simulink model "Audio_BPSK"  (R2021b)
settings: Solver=VariableStepAuto  StartTime=0.0  StopTime=2  RelTol=1e-3
model workspace (MAT data in the model file):
  Fcarrier = 8000
  Fsampling = 48000
  Tsymbol = 0.0005
  beta = 0.5
  costas_alpha = 0.1
  costas_coeffs = [0.078989 0.085868 0.091518 0.095721 0.098311 0.099186 0.098311 0.095721 0.09151 0.085868 0.078989]
  filterSpan = 2
  gardner_Ki = -0.000314099
  gardner_Kp = -0.0282632
  int_presc = 0.6
  preamble = [1 1 1 -1 1]
  preambleLength = 5
  samplesPerSymbol = 24
  symbolsPerFrame = 8
undefined symbols (not defined in the file or in its folder): doppler, fdesignblkfcn, gcbh
libraries: commutil2 x3, commfilt2 x2, simulink x1, commsink2 x1, impairlib x1, commrandsrc3 x1, commchan3 x1
settings Model: SimulationMode=accelerator  PacingRate=0.071000  Creator=asiem  LastModifiedBy=asiem

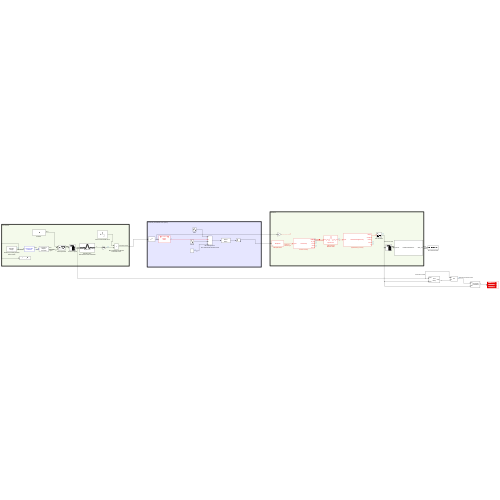
[thumbnail: Simulink's stored preview of the top-level diagram]
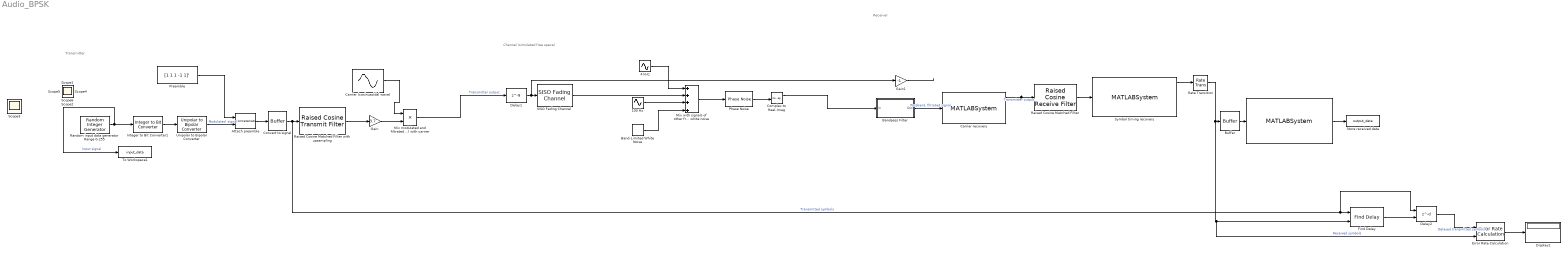
== system Audio_BPSK ==
  note: Receiver
  note: Channel (simulated free space)
  note: Transmitter
  " " : MATLABSystem  System=DataFramesDetector  buffer_length=512  preamble=[ 1, 1, 1, -1, 1 ]  data_frames_length=8  SimulateUsing=Interpreted execution
      mask Type: DataFramesDetector
      mask Display:
      | disp('DataFramesDetector');
      | port_label('input',1,'symbols');
      | port_label('output',1,'data_out');
  100 Hz : Sin  Amplitude=0.6  Bias=0.120  Frequency=100*2*pi  Phase=3*pi/4  SampleTime=1/48000
  "4 kHz " : Sin  Amplitude=0.3  Frequency=3000*2*pi  Phase=pi/3  SampleTime=1/48000
  Attach preamble : Concatenate  Mode=Multidimensional array
  Band-Limited White Noise : simulink/Sources/Band-Limited White Noise  Cov=[0.00000005]  Ts=1/Fsampling  seed=[23341]
  Bandpass Filter : Subsystem  DialogController=fdesignblkfcn  InitFcn=fdesignblkfcn(gcbh, {'InitFcn'});  mask(Bandpass Filter){}
      mask help: Design a bandpass filter
      settings: CopyFcn=fdesignblkfcn(gcbh, {'CopyFcn'});
      mask Help: helpview(mapfilelocation('dsp'), 'dspbandpassfilter');
      mask Display: disp('Bandpass');
  Buffer : Buffer  N=512  OutputFrames=off
  Carrier (cosinusoidal wave) : Sin  Frequency=Fcarrier*2*pi  Phase=pi/2 + pi/3  SampleTime=1/Fsampling
  Carrier recovery : MATLABSystem  System=CostasLoop  alpha=costas_alpha  beta=costas_alpha * costas_alpha / 4  lpf_coeffs=costas_coeffs  Fc=Fcarrier  Fs=Fsampling  REF_PERIOD=1e6 / Fcarrier  SAMPLE_PERIOD=1e6 / Fsampling  intgralf=int_presc * costas_alpha / (1e6 / Fcarrier)  SimulateUsing=Interpreted execution
      mask Type: CostasLoop
      mask Display:
      | disp('CostasLoop');
      | port_label('input',1,'input');
      | port_label('output',1,'S_I');
      | port_label('output',2,'S_Q');
      | port_label('output',3,'lock');
      | port_label('output',4,'ask');
      | port_label('output',5,'error');
  Complex to Real-Imag : ComplexToRealImag
  Convert to signal : Buffer  N=1  OutputFrames=off
  Delay1 : Delay  DelayLength=9  InputProcessing=Columns as channels (frame based)
  Delay2 : Delay  DelayLengthSource=Input port  DelayLength=3  InputProcessing=Columns as channels (frame based)
      settings: InputPortMap=u0,p1
  Display2 : Display
  Error Rate Calculation : commsink2/Error Rate Calculation  N=0  st_delay=0  cp_mode=Entire frame  subframe=[]  PMode=Port  WsName=ErrorVec  RsMode2=off  stop=off  numErr=100  maxBits=1e6
  Find Delay : commutil2/Find Delay  corrLength=20  chgSigOP=off  stopUpdate=off  numConstDelay=3
      settings: SourceProductBaseCode=CM
  Gain : Gain  Gain=3.7
  Gain1 : Gain  Gain=-1
  Integer to Bit Converter1 : commutil2/Integer to Bit Converter  nbits=symbolsPerFrame  signedInputValues=Unsigned  bitOrder=MSB first  outDtype=Inherit via internal rule
  Mix modulated and filtrated signal with carrier : Product
  Mix with signals of other frequencies and white noise : Sum  Inputs=++++
  Phase Noise : impairlib/Phase Noise  Level=-25  FrequencyOffset=3  SampleRate=Fsampling  RandomStream=mt19937ar with seed  Seed=32  SimulateUsing=Interpreted execution
      settings: SourceProductBaseCode=CM,AM,SX
  Preamble : Constant  Value=[1 1 1 -1 1]'  VectorParams1D=off
  "Raised Cosine Matched Filter " : commfilt2/Raised Cosine Receive Filter  filtType=Square root  R=beta  filtSpan=filterSpan  N=samplesPerSymbol  downFactor=1  downOffset=0  filterGain=1/2  InputProcessing=Columns as channels (frame based)  RateOptions=Allow multirate processing  framing=Mute  checkCoeff=on  variableName=rcRxFilt  currentFiltSpan=10  D=5  inputOffset=0  sampMode=Mute  saveAsFlag=0  rateMode=Downsampling  checkGain=Normalized  launchFVT=on  roundingMode=Floor  overflowMode=off  coeffDataTypeStr=Inherit: Same word length as input  coeffMin=[]  coeffMax=[]  coeffLastDataTypeStr=Inherit: Same word length as input  accumDataTypeStr=Inherit: Same as product output  accumLastDataTypeStr=Inherit: Same as product output  outputDataTypeStr=Inherit: Same as accumulator  outputMin=[]  outputMax=[]  outputLastDataTypeStr=Inherit: Same as accumulator
  Raised Cosine Matched Filter with upsampling : commfilt2/Raised Cosine Transmit Filter  filtType=Square root  R=beta  filtSpan=filterSpan  N=samplesPerSymbol  filterGain=1  InputProcessing=Columns as channels (frame based)  RateOptions=Allow multirate processing  framing=Mute  checkCoeff=on  variableName=rcTxFilt  checkGain=Normalized  sampMode=Mute  saveAsFlag=0  currentFiltSpan=10  D=(10)/2  launchFVT=on  roundingMode=Floor  overflowMode=off  coeffDataTypeStr=Inherit: Same word length as input  coeffMin=[]  coeffMax=[]  coeffLastDataTypeStr=Inherit: Same word length as input  outputDataTypeStr=Inherit: Same as accumulator  outputMin=[]  outputMax=[]  outputLastDataTypeStr=Inherit: Same as accumulator
  Random input data generator Range 0-255 : commrandsrc3/Random Integer Generator  SetSize=2^symbolsPerFrame - 1  SeedSource=Auto  Seed=0  SampleTime=Tsymbol*(symbolsPerFrame+preambleLength)  SamplesPerFrame=1  OutputDataType=double  SimulateUsing=Interpreted execution
  "Rate Transition " : RateTransition  OutPortSampleTime=samplesPerSymbol/Fsampling
  SISO Fading Channel : commchan3/SISO Fading Channel  InheritSampleRate=on  SampleRate=1  PathDelays=[0 0.0016 0.0097 0.0131]  AveragePathGains=[0 -10 -15 -20]  NormalizePathGains=on  FadingDistribution=Rician  KFactor=7  DirectPathDopplerShift=0.01  DirectPathInitialPhase=0  MaximumDopplerShift=0.1  DopplerSpectrum=doppler('Jakes')  RandomStream=mt19937ar with seed  Seed=73  PathGainsOutputPort=off  ChannelFilterDelayOutputPort=off  SimulateUsing=Interpreted execution  Visualization=Impulse response  PathsForDopplerDisplay=1  SamplesToDisplay=100%
  "Store received data " : ToWorkspace  VariableName=output_data  SaveFormat=Structure  SampleTime=-1
  Symbol timing recovery : MATLABSystem  System=GardnerTimingRecovery  Kp=gardner_Kp  Ki=gardner_Ki  samplesPerBit=samplesPerSymbol  SimulateUsing=Interpreted execution
      mask Type: GardnerTimingRecovery
      mask Display:
      | disp('GardnerTimingRecovery');
      | port_label('input',1,'input');
      | port_label('output',1,'output');
      | port_label('output',2,'sample');
      | port_label('output',3,'index');
      | port_label('output',4,'error');
      | port_label('output',5,'v');
  To Workspace1 : ToWorkspace  VariableName=input_data  SampleTime=-1
      settings: Save2DSignal=2-D array (concatenate along first dimension)
  Unipolar to Bipolar Converter : commutil2/Unipolar to Bipolar Converter  M=2  polarity=Positive  dataType=Inherit via internal rule
  Scope{,1..6} (7 alike) : Scope
  wires:
  Carrier (cosinusoidal wave)/1 -> Mix modulated and filtrated signal with carrier/1
  Mix modulated and filtrated signal with carrier/1 -> Delay1/1  "Transmitter output"
  Random input data generator Range 0-255/1 -> To Workspace1/1, Integer to Bit Converter1/1  "Input signal"
  Integer to Bit Converter1/1 -> Unipolar to Bipolar Converter/1
  Preamble/1 -> Attach preamble/1
  Unipolar to Bipolar Converter/1 -> Attach preamble/2  "Modulated  signal"
  Attach preamble/1 -> Convert to signal/1
  Raised Cosine Matched Filter with upsampling/1 -> Gain/1
  "Raised Cosine Matched Filter "/1 -> Symbol timing recovery/1
  "4 kHz "/1 -> Mix with signals of other frequencies and white noise/1
  100 Hz/1 -> Mix with signals of other frequencies and white noise/3
  Symbol timing recovery/1 -> "Rate Transition "/1
  Band-Limited White Noise/1 -> Mix with signals of other frequencies and white noise/4
  "Rate Transition "/1 -> Error Rate Calculation/2, Find Delay/2, Buffer/1  "Received symbols"
  Convert to signal/1 -> Delay2/1, Find Delay/1, Raised Cosine Matched Filter with upsampling/1  "Transmitted symbols"
  Error Rate Calculation/1 -> Display2/1
  Delay2/1 -> Error Rate Calculation/1  "Delayed transmitted symbols"
  Find Delay/1 -> Delay2/2
  Gain/1 -> Mix modulated and filtrated signal with carrier/2
  Mix with signals of other frequencies and white noise/1 -> Phase Noise/1
  Buffer/1 -> " "/1
  " "/1 -> "Store received data "/1
  Complex to Real-Imag/1 -> Bandpass Filter/1(In)
  Delay1/1 -> SISO Fading Channel/1, Gain1/1
  Phase Noise/1 -> Complex to Real-Imag/1
  SISO Fading Channel/1 -> Mix with signals of other frequencies and white noise/2
  Carrier recovery/1 -> "Raised Cosine Matched Filter "/1  "Transmitter output"
  Bandpass Filter/1(Out) -> Carrier recovery/1  "Passband, filtrated signal"
  Gain1/1 -> ?

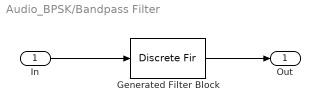
== system Audio_BPSK/Bandpass Filter ==
  In : Inport
  Generated Filter Block : DiscreteFir  Tag=BlockMethodSubSystem  FilterStructure=Direct form symmetric  Coefficients=[0.0181921898927299361 4.69418855769848753e-05 -0.0106776564766215953 -0.00561031340470226608 4.95844029183965844e-07 -0.00701295998675918481 -0.0143928598868380431 -4.78431862282031287e-05 0.0305474288818812813 0.0391734106943500138 8.00942445870862302e-05 -0.0563294270782706413 -0.0647524300822733961 -8.70136472838366529e-05 0.0799358227411005456 0.0866307974123829011 6.63896436749199958e-05 -0.0970625700450543222 -0.100766774960784553 -2.47420235520264227e-05 0.104480480530872971 0.104480480530872971 -2.47420235520264227e-05 -0.100766774960784553 -0.0970625700450543222 6.63896436749199958e-05 0.0866307974123829011 0.0799358227411005456 -8.70136472838366529e-05 -0.0647524300822733961 -0.0563294270782706413 8.00942445870862302e-05 0.0391734106943500138 0.0305474288818812813 -4.78431862282031287e-05 -0.0143928598868380431 -0.00701295998675918481 4.95844029183965844e-07 -0.00561031340470226608 -0.0106776564766215953 4.69418855769848753e-05 0.0181921898927299361]  InputProcessing=Columns as channels (frame based)
  Out : Outport  VectorParamsAs1DForOutWhenUnconnected=off
  wires:
  In/1 -> Generated Filter Block/1
  Generated Filter Block/1 -> Out/1
